simulink model "testbench_with_kalman_filter"  (R2016a)
settings: Solver=FixedStepAuto  StartTime=0.0  StopTime=10.0  RelTol=1e-3
values from neighbouring files (symbols this model uses):
  A = [1 1 0;0 1 1;0 0 1]    [kalman_script.m]
undefined symbols (not defined in the file or in its folder): Discrete, Time
libraries: legoev3lib x2, simulink x2, ctrlSharedLib x1
settings Model: SimulationMode=external  ExtModeTrigDuration=2  Creator=Shobhit  LastModifiedBy=Shobhit
settings SolverCC: PositivePriorityOrder=on
settings OptimizationCC: OptimizeModelRefInitCode=on  LifeSpan=1  MaxStackSize=64
settings DebuggingCC: AlgebraicLoopMsg=none
settings HardwareCC: ProdBitPerPointer=32  ProdLargestAtomicInteger=Long  ProdWordSize=32  ProdHWDeviceType=ARM Compatible->ARM 9  UseEmbeddedCoderFeatures=off  UseSimulinkCoderFeatures=off
settings RTWCC: SystemTargetFile=ert.tlc  HardwareBoard=LEGO MINDSTORMS EV3  TemplateMakefile=ert_default_tmf  GenerateReport=on  Toolchain=Sourcery G++ Lite v2009q3  IncludeHyperlinkInReport=on  LaunchReport=on  GenerateTraceInfo=on  GenerateTraceReport=on  GenerateTraceReportSl=on  GenerateTraceReportSf=on  GenerateTraceReportEml=on
settings CodeAppCC: ForceParamTrailComments=on  IgnoreCustomStorageClasses=off  OperatorAnnotations=on  SimulinkDataObjDesc=on  SFDataObjDesc=on  MATLABFcnDesc=on  InsertBlockDesc=on  MATLABSourceComments=on
settings ERTTargetCC: SupportContinuousTime=on  SupportNonInlinedSFcns=on  SupportVariableSizeSignals=on

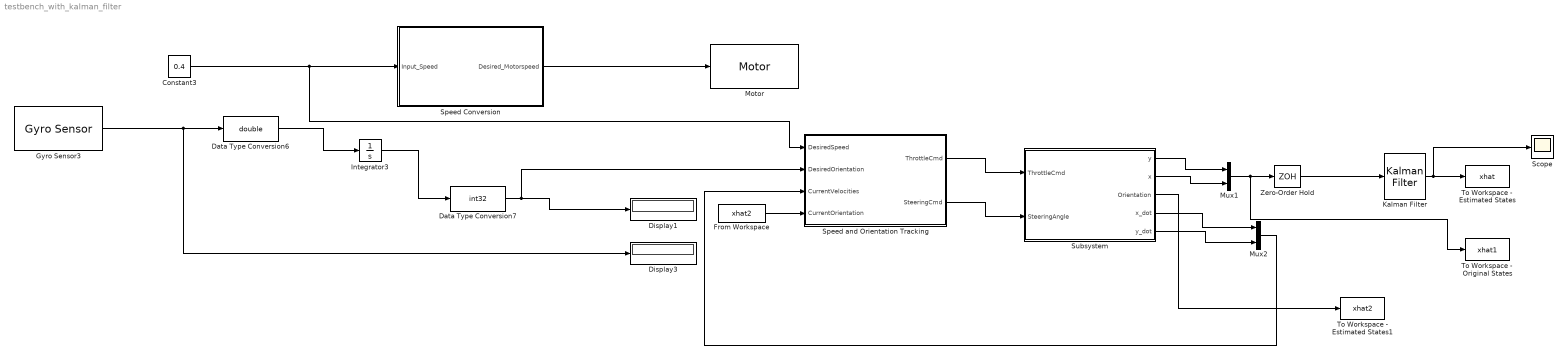
== system testbench_with_kalman_filter ==
  Constant3 : Constant  Value=0.4
  Data Type Conversion6 : DataTypeConversion  OutDataTypeStr=double  RndMeth=Ceiling
  Data Type Conversion7 : DataTypeConversion  OutDataTypeStr=int32  RndMeth=Ceiling
  Display1 : Display
  Display3 : Display
  From Workspace : FromWorkspace  VariableName=xhat2  SampleTime=0
  Gyro Sensor3 : legoev3lib/Gyro Sensor  portNumber=2  sampleTime=0.1
  Integrator3 : Integrator
  Kalman Filter : ctrlSharedLib/Kalman Filter  TimeDomain=Discrete-Time  UseCurrentEstimator=on  ModelSource=Individual A, B, C, D matrices  ModelSourceVariable=sys  A=A  B=1  C=[1 0 0;0 0 1]  D=0  NumberOfStates=1  NumberOfInputs=1  NumberOfOutputs=1  InitialEstimateSource=Dialog  X0=0  P0=10  UseK=off  UseGH=off  NumberOfProcessNoiseInputs=1  G=1  TimeInvariantG=on  H=0  TimeInvariantH=on  Q=0.05  TimeInvariantQ=on  R=10  TimeInvariantR=on  N=0  TimeInvariantN=on  AddInputPort=off  AddEnablePort=off  OutputEstimatedY=off  OutputP=off  Ts=-1
  Motor : legoev3lib/Motor  sportNumber=A  sstopAction=Brake
  Mux1 : Mux  Inputs=2
  Mux2 : Mux  Inputs=2
  Scope : Scope
  Speed Conversion : Subsystem
  "Speed and Orientation Tracking " : Subsystem
  Subsystem : Subsystem
  To Workspace - Estimated States : ToWorkspace  VariableName=xhat  SampleTime=-1
      settings: Save2DSignal=2-D array (concatenate along first dimension)
  To Workspace - Estimated States1 : ToWorkspace  VariableName=xhat2  SampleTime=-1
      settings: Save2DSignal=2-D array (concatenate along first dimension)
  "To Workspace - Original States " : ToWorkspace  VariableName=xhat1  SampleTime=-1
      settings: Save2DSignal=2-D array (concatenate along first dimension)
  Zero-Order Hold : ZeroOrderHold
  wires:
  Integrator3/1 -> Data Type Conversion7/1
  Data Type Conversion6/1 -> Integrator3/1
  Gyro Sensor3/1 -> Display3/1, Data Type Conversion6/1
  Speed Conversion/1(Desired_Motorspeed) -> Motor/1
  "Speed and Orientation Tracking "/1(ThrottleCmd) -> Subsystem/1(ThrottleCmd)
  "Speed and Orientation Tracking "/2(SteeringCmd) -> Subsystem/2(SteeringAngle)
  Subsystem/4("x_dot ") -> Mux2/1
  Subsystem/5(y_dot) -> Mux2/2
  Mux2/1 -> "Speed and Orientation Tracking "/3(CurrentVelocities)
  Subsystem/2(x) -> Mux1/2
  Subsystem/1(y) -> Mux1/1
  Mux1/1 -> "To Workspace - Original States "/1, Zero-Order Hold/1
  Zero-Order Hold/1 -> Kalman Filter/1
  Kalman Filter/1 -> Scope/1, To Workspace - Estimated States/1
  Constant3/1 -> "Speed and Orientation Tracking "/1(DesiredSpeed), Speed Conversion/1(Input_Speed)
  Data Type Conversion7/1 -> "Speed and Orientation Tracking "/2(DesiredOrientation), Display1/1
  Subsystem/3("Orientation ") -> To Workspace - Estimated States1/1
  From Workspace/1 -> "Speed and Orientation Tracking "/4(CurrentOrientation)

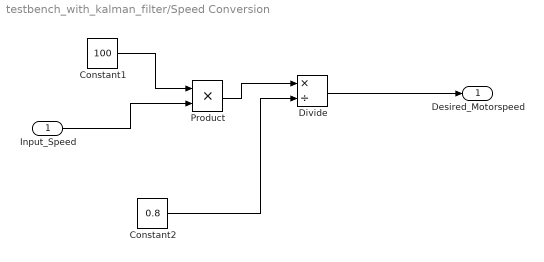
== system testbench_with_kalman_filter/Speed Conversion ==
  Input_Speed : Inport
  Constant1 : Constant  Value=100
  Constant2 : Constant  Value=0.8
  Divide : Product  Inputs=*/
  Product : Product
  Desired_Motorspeed : Outport
  wires:
  Divide/1 -> Desired_Motorspeed/1
  Input_Speed/1 -> Product/2
  Constant2/1 -> Divide/2
  Product/1 -> Divide/1
  Constant1/1 -> Product/1

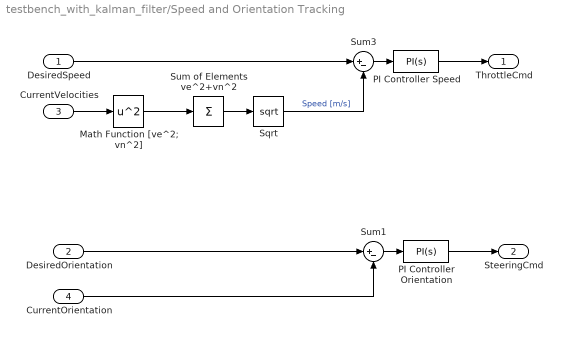
== system testbench_with_kalman_filter/Speed and Orientation Tracking  ==
  DesiredSpeed : Inport
  DesiredOrientation : Inport  Port=2
  CurrentVelocities : Inport  Port=3
  CurrentOrientation : Inport  Port=4
  Math Function [ve^2; vn^2] : Math  Operator=square  SaturateOnIntegerOverflow=on
  PI Controller Orientation : simulink/Continuous/PID Controller  Controller=PI  TimeDomain=Continuous-time  SampleTime=-1  IntegratorMethod=Forward Euler  FilterMethod=Forward Euler  Form=Parallel  UseFilter=on  ControllerParametersSource=internal  P=1  I=0.3  D=0  N=100  InitialConditionSource=internal  InitialConditionForIntegrator=0  InitialConditionForFilter=0  ExternalReset=none  LimitOutput=on  UpperSaturationLimit=20  LowerSaturationLimit=-20  LinearizeAsGain=off  AntiWindupMode=clamping  Kb=1  TrackingMode=off  Kt=1  PParamMin=[]  PParamMax=[]  IParamMin=[]  IParamMax=[]  DParamMin=[]  DParamMax=[]  NParamMin=[]  NParamMax=[]  KbParamMin=[]  KbParamMax=[]  KtParamMin=[]  KtParamMax=[]  POutMin=[]  POutMax=[]  IOutMin=[]  IOutMax=[]  DOutMin=[]  DOutMax=[]  NOutMin=[]  NOutMax=[]  KbOutMin=[]  KbOutMax=[]  KtOutMin=[]  KtOutMax=[]  IntegratorOutMin=[]  IntegratorOutMax=[]  FilterOutMin=[]  FilterOutMax=[]  SumOutMin=[]  SumOutMax=[]  SumI1OutMin=[]  SumI1OutMax=[]  SumI2OutMin=[]  SumI2OutMax=[]  SumI3OutMin=[]  SumI3OutMax=[]  SumDOutMin=[]  SumDOutMax=[]  SaturationOutMin=[]  SaturationOutMax=[]  IntegratorContinuousStateAttributes=''  IntegratorStateMustResolveToSignalObject=off  IntegratorRTWStateStorageClass=Auto  FilterContinuousStateAttributes=''  FilterStateMustResolveToSignalObject=off  FilterRTWStateStorageClass=Auto  DifferentiatorICPrevScaledInput=0  DifferentiatorOutMin=[]  DifferentiatorOutMax=[]
  PI Controller Speed : simulink/Continuous/PID Controller  Controller=PI  TimeDomain=Continuous-time  SampleTime=-1  IntegratorMethod=Forward Euler  FilterMethod=Forward Euler  Form=Parallel  UseFilter=on  ControllerParametersSource=internal  P=0.15  I=0.01  D=0  N=100  InitialConditionSource=internal  InitialConditionForIntegrator=0  InitialConditionForFilter=0  ExternalReset=none  LimitOutput=on  UpperSaturationLimit=1  LowerSaturationLimit=-1  LinearizeAsGain=off  AntiWindupMode=clamping  Kb=1  TrackingMode=off  Kt=1  PParamMin=[]  PParamMax=[]  IParamMin=[]  IParamMax=[]  DParamMin=[]  DParamMax=[]  NParamMin=[]  NParamMax=[]  KbParamMin=[]  KbParamMax=[]  KtParamMin=[]  KtParamMax=[]  POutMin=[]  POutMax=[]  IOutMin=[]  IOutMax=[]  DOutMin=[]  DOutMax=[]  NOutMin=[]  NOutMax=[]  KbOutMin=[]  KbOutMax=[]  KtOutMin=[]  KtOutMax=[]  IntegratorOutMin=[]  IntegratorOutMax=[]  FilterOutMin=[]  FilterOutMax=[]  SumOutMin=[]  SumOutMax=[]  SumI1OutMin=[]  SumI1OutMax=[]  SumI2OutMin=[]  SumI2OutMax=[]  SumI3OutMin=[]  SumI3OutMax=[]  SumDOutMin=[]  SumDOutMax=[]  SaturationOutMin=[]  SaturationOutMax=[]  IntegratorContinuousStateAttributes=''  IntegratorStateMustResolveToSignalObject=off  IntegratorRTWStateStorageClass=Auto  FilterContinuousStateAttributes=''  FilterStateMustResolveToSignalObject=off  FilterRTWStateStorageClass=Auto  DifferentiatorICPrevScaledInput=0  DifferentiatorOutMin=[]  DifferentiatorOutMax=[]
  Sqrt : Sqrt  SaturateOnIntegerOverflow=on
  Sum of Elements ve^2+vn^2 : Sum  Inputs=+
  Sum1 : Sum  Inputs=|+-
  Sum3 : Sum  Inputs=|+-
  ThrottleCmd : Outport
  SteeringCmd : Outport  Port=2
  wires:
  PI Controller Speed/1 -> ThrottleCmd/1
  DesiredSpeed/1 -> Sum3/1
  Sum3/1 -> PI Controller Speed/1
  Math Function [ve^2; vn^2]/1 -> Sum of Elements ve^2+vn^2/1
  CurrentVelocities/1 -> Math Function [ve^2; vn^2]/1
  Sum of Elements ve^2+vn^2/1 -> Sqrt/1
  Sqrt/1 -> Sum3/2  "Speed [m/s]"
  DesiredOrientation/1 -> Sum1/1
  PI Controller Orientation/1 -> SteeringCmd/1
  Sum1/1 -> PI Controller Orientation/1
  CurrentOrientation/1 -> Sum1/2

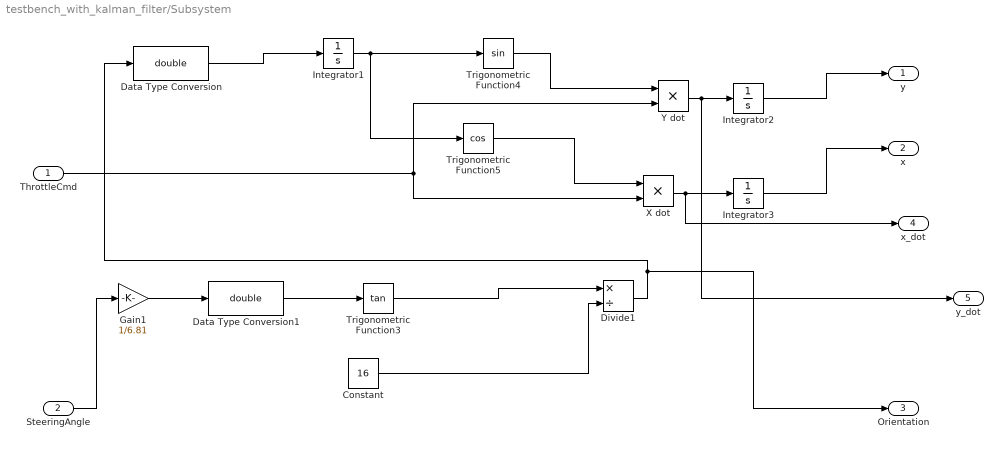
== system testbench_with_kalman_filter/Subsystem ==
  ThrottleCmd : Inport
  SteeringAngle : Inport  Port=2
  Constant : Constant  Value=16
  Data Type Conversion : DataTypeConversion  OutDataTypeStr=double
  Data Type Conversion1 : DataTypeConversion  OutDataTypeStr=double
  Divide1 : Product  Inputs=*/
  Gain1 : Gain  Gain=1/6.81
  Integrator1 : Integrator
  Integrator2 : Integrator
  Integrator3 : Integrator
  Trigonometric Function3 : Trigonometry  Operator=tan  OutputSignalType=real
  Trigonometric Function4 : Trigonometry
  Trigonometric Function5 : Trigonometry  Operator=cos
  "X dot " : Product
  "Y dot " : Product
  y : Outport
  x : Outport  Port=2
  "Orientation " : Outport  Port=3
  "x_dot " : Outport  Port=4
  y_dot : Outport  Port=5
  wires:
  Gain1/1 -> Data Type Conversion1/1
  Integrator1/1 -> Trigonometric Function5/1, Trigonometric Function4/1
  ThrottleCmd/1 -> "X dot "/2, "Y dot "/2
  Trigonometric Function5/1 -> "X dot "/1
  Trigonometric Function4/1 -> "Y dot "/1
  "X dot "/1 -> "x_dot "/1, Integrator3/1
  "Y dot "/1 -> y_dot/1, Integrator2/1
  Data Type Conversion/1 -> Integrator1/1
  Integrator2/1 -> y/1
  Integrator3/1 -> x/1
  SteeringAngle/1 -> Gain1/1
  Data Type Conversion1/1 -> Trigonometric Function3/1
  Trigonometric Function3/1 -> Divide1/1
  Constant/1 -> Divide1/2
  Divide1/1 -> "Orientation "/1, Data Type Conversion/1
